simulink model "joint_calibrator"  (R2016a)
settings: Solver=VariableStepAuto  StartTime=0.0  StopTime=10.0  RelTol=1e-3
undefined symbols (not defined in the file or in its folder): Hip_HAA
libraries: xpcethercatlib x5
settings Model: Creator=tech  LastModifiedBy=tech

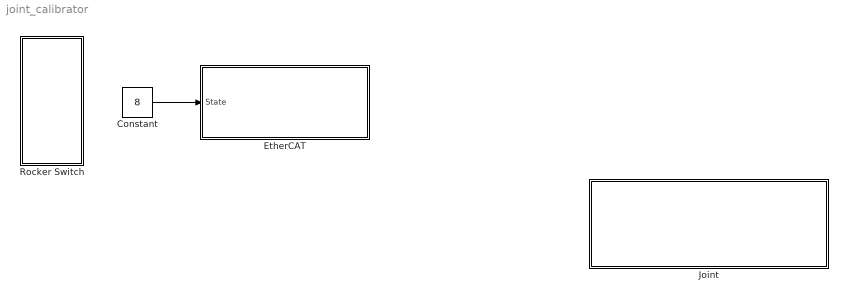
== system joint_calibrator ==
  Constant : Constant  Value=8
  EtherCAT : Subsystem
  Joint : Subsystem
  Rocker Switch : Subsystem  DialogController=hmiCreateDDGDialog  IsWebBlock=on  mask(MWDashboardBlock){webBlockId=cc82a37f-2998-4a3d-a0a0-1cb750b10d1a, webBlockType=rockerswitch, ShowInLibBrowser=on, ShowInitialText=on, HMISrcModelName=joint_calibrator}
      mask prompts: webBlockId "WebBlock Id"; webBlockType "WebBlock Type"; HMISrcModelName "Source Model"
      mask Help: helpview([docroot '/mapfiles/simulink.map'], 'hmi_rocker_switch')
      mask Display:
      | if strcmp(get_param(bdroot(gcb),'BlockDiagramType'), 'library')
      |     image([(matlabroot) '/toolbox/simulink/hmi/icons/RockerSwitch.png']);
      | end
  wires:
  Constant/1 -> EtherCAT/1(State)

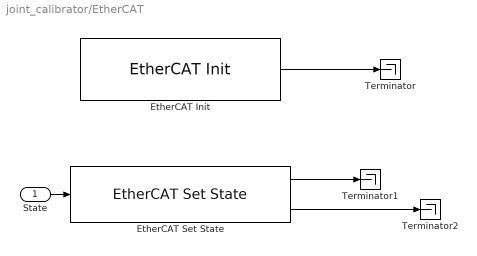
== system joint_calibrator/EtherCAT ==
  State : Inport
  "EtherCAT Init " : xpcethercatlib/EtherCAT Init   Priority=0  config_file=C:\Software\MATLAB\simulink-models\EtherCAT Config files\full_setup_v1.0.xml  device_id=0  pci_bus=2  pci_slot=0  dctuning=1  enaDebug=off  enaDC=on  errLink=off  masterDbg=off  stateChgDbg=off  baseClock=off  masterCfg=off  logFile='c:\dbglog.txt'  sample_time=0.001000
  "EtherCAT Set State " : xpcethercatlib/EtherCAT Set State   device_id=0  timeout=0  sample_time=0
  Terminator : Terminator
  Terminator1 : Terminator
  Terminator2 : Terminator
  wires:
  "EtherCAT Init "/1 -> Terminator/1
  "EtherCAT Set State "/2 -> Terminator2/1
  "EtherCAT Set State "/1 -> Terminator1/1
  State/1 -> "EtherCAT Set State "/1

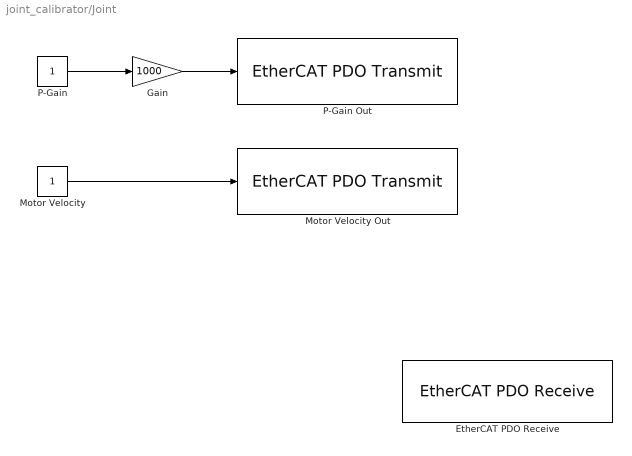
== system joint_calibrator/Joint ==
  EtherCAT PDO Receive : xpcethercatlib/EtherCAT PDO Receive  Priority=2  sig_name=Hip_HAA.Inputs.L_crutchForce[0]  sig_offset=336  sig_type=int32  type_size=32  sig_dim=1  device_id=0  sample_time=0.001
  Gain : Gain  Gain=1000
  Motor Velocity : Constant
  Motor Velocity Out : xpcethercatlib/EtherCAT PDO Transmit   Priority=3  sig_name=Hip_HAA.Outputs.L_velocitySetPoint  sig_offset=1432  sig_type=int16  type_size=16  sig_dim=1  device_id=0  sample_time=0.001
  P-Gain : Constant
  P-Gain Out : xpcethercatlib/EtherCAT PDO Transmit   Priority=3  sig_name=Hip_HAA.Outputs.L_data[0]  sig_offset=1960  sig_type=int32  type_size=32  sig_dim=1  device_id=0  sample_time=0.001
  wires:
  Motor Velocity/1 -> Motor Velocity Out/1
  Gain/1 -> P-Gain Out/1
  P-Gain/1 -> Gain/1

== system joint_calibrator/Rocker Switch ==
